simulink model "SG__REF_I_135_1to8"  (R2022b)
settings: Solver=FixedStepAuto  StartTime=0.0  StopTime=Inf  RelTol=1e-3  EnableMultiTasking=on
model workspace (MAT data in the model file):
  N_trig = Simulink.Parameter
  N_trig.Value = 4
  N_trig.Description = 'number of samples for triggered pulse for recording'
  N_trig.DataType = 'auto'
  N_trig.Complexity = 'real'
  N_trig.Dimensions = [1 1]
  a_1 = Simulink.Parameter
  a_1.Value = [1 1 1]
  a_1.DataType = 'auto'
  a_1.Complexity = 'real'
  a_1.Dimensions = [1 3]
  b_1 = Simulink.Parameter
  b_1.Value = [0.5 0.5 0.5]
  b_1.DataType = 'auto'
  b_1.Complexity = 'real'
  b_1.Dimensions = [1 3]
  enable_source = Simulink.Parameter
  enable_source.Value = 0
  enable_source.DataType = 'boolean'
  enable_source.Complexity = 'real'
  enable_source.Dimensions = [1 1]
  freq_fin = Simulink.Parameter
  freq_fin.Value = 1200
  freq_fin.DataType = 'auto'
  freq_fin.Complexity = 'real'
  freq_fin.Dimensions = [1 1]
  freq_ini = Simulink.Parameter
  freq_ini.Value = 150
  freq_ini.DataType = 'auto'
  freq_ini.Complexity = 'real'
  freq_ini.Dimensions = [1 1]
  k_1 = Simulink.Parameter
  k_1.Value = [0 0 0]
  k_1.DataType = 'auto'
  k_1.Complexity = 'real'
  k_1.Dimensions = [1 3]
  rec = Simulink.Parameter
  rec.Value = 0
  rec.DataType = 'boolean'
  rec.Complexity = 'real'
  rec.Dimensions = [1 1]
  src_select = Simulink.Parameter
  src_select.Value = 0
  src_select.DataType = 'auto'
  src_select.Complexity = 'real'
  src_select.Dimensions = [1 1]
  sweep_gain = Simulink.Parameter
  sweep_gain.Value = 0.02
  sweep_gain.DataType = 'auto'
  sweep_gain.Complexity = 'real'
  sweep_gain.Dimensions = [1 1]
  tmax = Simulink.Parameter
  tmax.Value = 10
  tmax.DataType = 'auto'
  tmax.Complexity = 'real'
  tmax.Dimensions = [1 1]
  ts_rec = Simulink.Parameter
  ts_rec.Value = 0.0001
  ts_rec.DataType = 'auto'
  ts_rec.Complexity = 'real'
  ts_rec.Dimensions = [1 1]
libraries: simulink x3, speedgoatlib_IO135 x2, hdlsllib x2, slrealtimeloglib x1, slrealtimetgmanagement x1
settings Model: SimulationMode=external  DataflowThreadingImplementation=Pthreads  Creator=padlewsk  LastModifiedBy=padlewsk
settings SolverCC: ConcurrentTasks=on  AlgebraicLoopSolver=TrustRegion  PositivePriorityOrder=on  AutoInsertRateTranBlk=on
settings DataIOCC: SaveFormat=StructureWithTime
settings OptimizationCC: GainParamInheritBuiltInType=on  RollThreshold=9  EfficientFloat2IntCast=on  SimCompilerOptimization=on
settings DebuggingCC: TasksWithSamePriorityMsg=none  UnconnectedInputMsg=warning  UnconnectedOutputMsg=warning  UnconnectedLineMsg=warning
settings HardwareCC: ProdBitPerLong=64  ProdLongLongMode=on  ProdHWDeviceType=Intel->x86-64 (Linux 64)
settings ModelReferenceCC: EnableRefExpFcnMdlSchedulingChecks=on  ModelReferenceNumInstancesAllowed=Single
settings RTWCC: Description=Simulink Real-Time  SystemTargetFile=slrealtime.tlc  TemplateMakefile=slrealtime_default_tmf  Toolchain=Simulink Real-Time Toolchain  BuildConfiguration=Faster Runs  CodeExecutionProfiling=on  TargetLang=C++

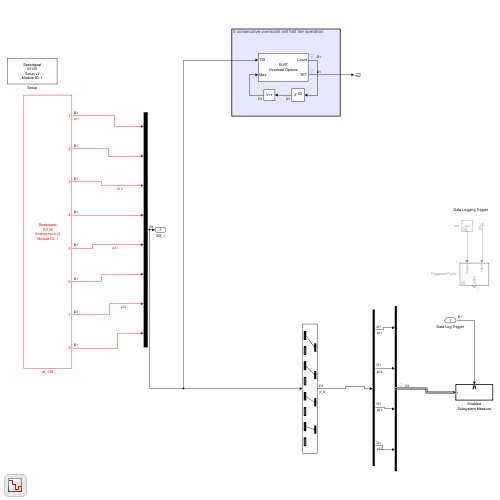
[thumbnail: Simulink's stored preview of the top-level diagram]
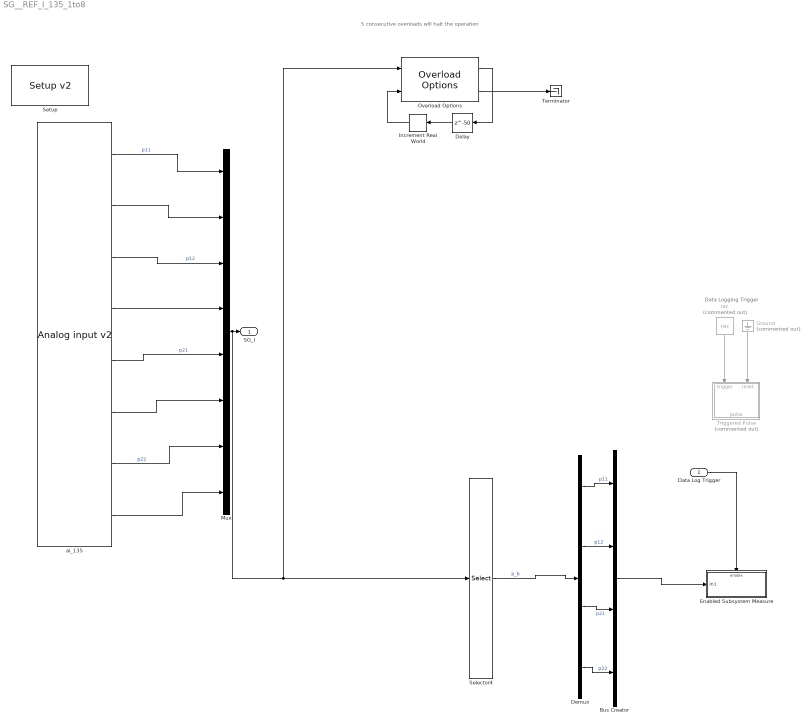
== system SG__REF_I_135_1to8 ==
  note: Data Logging Trigger
  note: 5 consecutive overloads will halt the operation
  Data Log Trigger : Inport  OutDataTypeStr=boolean
  Bus Creator : BusCreator  Inputs=4
  Delay : Delay  DelayLength=50
  Demux : Demux
  Enabled Subsystem Measure : Subsystem
  Ground : Ground  Commented=on
  Increment Real World : simulink/Additional Math & Discrete/Additional Math: Increment - Decrement/Increment Real World
  Mux : Mux  Inputs=8
  Overload Options : slrealtimetgmanagement/Overload Options  startupDur=1  startupDurSrc=Tunable Parameter  maxOverload=0  maxOverloadSrc=Input Port  TETFlag=on
  Selector4 : Selector  InputPortWidth=8  IndexOptions=Index vector (dialog)  Indices=[1:2:8]  OutputSizes=1
  Setup : speedgoatlib_IO135/Setup v2   parPciSlot=-1  parModuleId=1  parInterModuleSync=None  parConvClockBaseRate=60MHz  parConvClock1Divider=20000  parConvClock2Divider=20000  parFrameTriggerEnable=off  parFrameTriggerDivider=10  parConvClock1BaseRate=3  parConvClock2BaseRate=3  parFrameTriggerClock=1  parAdcChannels=[1:8]  parAdcRange1=+-5V  parAdcRange2=+-5V  parAdcRange3=+-5V  parAdcRange4=+-5V  parAdcVoltageRange=[1 1 1 1]  parAdcOversampling1=None  parAdcOversampling2=None  parAdcOversampling3=None  parAdcOversampling4=None  parAdcOversamplRate=[1 1 1 1]  parAdcAutoCorrection=on  parAdcContSampling=off  parAdcDmaEnable=off  parAdcDmaClock=Clock 1  parAdcFrameSize_=100  parAdcSampleTime_=-1  parAdcActiveDmaDevices=[1 1 1 1]  parAdcFrameTriggerEnable=0  parAdcFrameSize=100  parAdcSampleTime=0.0333333333333333  parDacChannels=[1:16]  parDacInitValues=0  parDacReset=1  parDacRange1=+-10V  parDacRange2=+-10V  parDacRange3=+-10V  parDacRange4=+-10V  parDacRange5=+-10V  parDacRange6=+-10V  parDacRange7=+-10V  parDacRange8=+-10V  parDacRange9=+-10V  parDacRange10=+-10V  parDacRange11=+-10V  parDacRange12=+-10V  parDacRange13=+-10V  parDacRange14=+-10V  parDacRange15=+-10V  parDacRange16=+-10V  parDacVoltageRange=[5 5 5 5 5 5 5 5 5 5 5 5 5 5 5 5]  parDacAutoCorrection=on  parDacSyncOut=off  parDacDmaEnable=off  parDacDmaLatency=Until next frame  parDacDmaClock=Clock 1  parDacFrameSize_=100  parDacSampleTime_=-1  parDacActiveDmaDevices=[1 1 1 1]  parDacFrameTriggerEnable=0  parDacFrameSize=100  parDacSampleTime=0.0333333333333333  parDoChannels=[]  parDoInitValues=0  parDoReset=1  parDiChannels=[]  parDiDebounceEnable=off  parDiDebounceTime=0  parDiDebounceValue=0  parDioPullRefFront=Pull-up 3.3V  parDioPullRefRear=Floating
      settings: SourceProductName=Simulink Real-Time: Speedgoat I/O Blockset
  Terminator : Terminator
  "Triggered Pulse " : Subsystem  Commented=on  TreatAsAtomicUnit=on  mask(Triggered Pulse){N=3000}
      mask prompts: N "Length (N samples)"
      mask help: Generates a single pulse of N samples length
  ai_135 : speedgoatlib_IO135/Analog input v2   parModuleId=1  parSampleTime=ts  parPciSlot=-1  parAdcChannels=[1 2 3 4 5 6 7 8]  parAdcVoltageRange=[1 1 1 1]  parAdcOversamplRate=[1 1 1 1]  parAdcContSampling=0  parAdcDmaEnable=0  parAdcActiveDmaDevices=[1 1 1 1]  parAdcFrameSize=100
      settings: SourceProductName=Simulink Real-Time: Speedgoat I/O Blockset
  rec : Constant  Commented=on  Value=rec  SampleTime=-1
  SG_I : Outport
  wires:
  ai_135/7 -> Mux/7  "p22"
  ai_135/2 -> Mux/2
  ai_135/8 -> Mux/8
  ai_135/4 -> Mux/4
  ai_135/5 -> Mux/5  "p21"
  ai_135/6 -> Mux/6
  ai_135/3 -> Mux/3  "p12"
  ai_135/1 -> Mux/1  "p11"
  Mux/1 -> Overload Options/1, Selector4/1, SG_I/1
  Demux/1 -> Bus Creator/1  "p11"
  Demux/2 -> Bus Creator/2  "p12"
  Demux/3 -> Bus Creator/3  "p21"
  Selector4/1 -> Demux/1  "p_b"
  rec/1 -> "Triggered Pulse "/1(trigger)
  Ground/1 -> "Triggered Pulse "/2(reset)
  Bus Creator/1 -> Enabled Subsystem Measure/1(In1)
  Data Log Trigger/1 -> Enabled Subsystem Measure/Enable
  Demux/4 -> Bus Creator/4  "p22"
  Delay/1 -> Increment Real World/1
  Increment Real World/1 -> Overload Options/2
  Overload Options/1 -> Delay/1
  Overload Options/2 -> Terminator/1

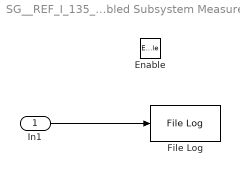
== system SG__REF_I_135_1to8/Enabled Subsystem Measure ==
  In1 : Inport
  Enable : EnablePort
  File Log : slrealtimeloglib/File Log  decimation=1  inputProcessing=Elements as channels (sample based)
  wires:
  In1/1 -> File Log/1

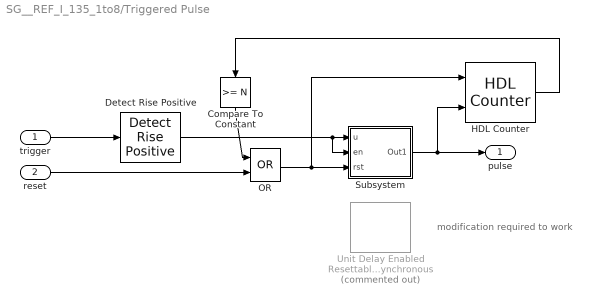
== system SG__REF_I_135_1to8/Triggered Pulse  ==
  note: modification required to work
  trigger : Inport
  reset : Inport  Port=2
  Compare To Constant : simulink/Logic and Bit Operations/Compare To Constant  relop=>=  const=N  OutDataTypeStr=boolean
  Detect Rise Positive : simulink/Logic and Bit Operations/Detect Rise Positive  vinit=0  OutDataTypeStr=boolean
  HDL Counter : hdlsllib/Sources/HDL Counter  CountType=Free running  CountInit=1  CountStep=1  CountMax=25  CountFromType=Initial value  CountFrom=1  CountResetPort=on  CountLoadPort=off  CountEnbPort=on  CountDirPort=off  CountHitOutputPort=off  CountDataType=Unsigned  CountWordLen=32  CountFracLen=0  CountSampTime=1
  OR : Logic  Operator=OR  AllPortsSameDT=off  OutDataTypeStr=boolean
  Subsystem : Subsystem
  Unit Delay Enabled Resettable Synchronous : hdlsllib/Discrete/Unit Delay Enabled Resettable Synchronous  Commented=on  InitialCondition=0.0  SampleTime=-1
  pulse : Outport  VectorParamsAs1DForOutWhenUnconnected=off
  wires:
  OR/1 -> Subsystem/3(rst), HDL Counter/1
  trigger/1 -> Detect Rise Positive/1
  Subsystem/1(Out1) -> HDL Counter/2, pulse/1
  Compare To Constant/1 -> OR/1
  reset/1 -> OR/2
  Detect Rise Positive/1 -> Subsystem/2(en), Subsystem/1(u)
  HDL Counter/1 -> Compare To Constant/1

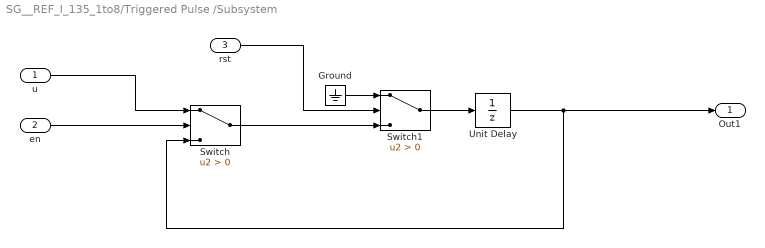
== system SG__REF_I_135_1to8/Triggered Pulse /Subsystem ==
  u : Inport
  en : Inport  Port=2
  rst : Inport  Port=3
  Ground : Ground
  Switch : Switch  Criteria=u2 > Threshold  SaturateOnIntegerOverflow=off  InputSameDT=off
  Switch1 : Switch  Criteria=u2 > Threshold  SaturateOnIntegerOverflow=off  InputSameDT=off
  Unit Delay : UnitDelay  SampleTime=-1  HasFrameUpgradeWarning=on
  Out1 : Outport
  wires:
  Unit Delay/1 -> Switch/3, Out1/1
  en/1 -> Switch/2
  u/1 -> Switch/1
  rst/1 -> Switch1/2
  Ground/1 -> Switch1/1
  Switch1/1 -> Unit Delay/1
  Switch/1 -> Switch1/3
